simulink model "coherent_demodulation"  (R2018b)
settings: Solver=VariableStepAuto  StartTime=0.0  StopTime=1  RelTol=1e-3
libraries: dsparch4 x2, commchan3 x1
settings Model: Creator=sangh  LastModifiedBy=sangh

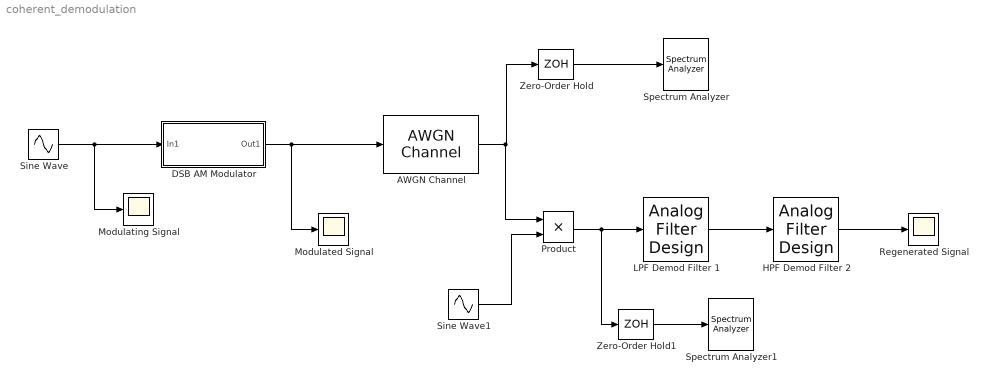
== system coherent_demodulation ==
  AWGN Channel : commchan3/AWGN Channel  InputProcessing=Columns as channels (frame based)  seed=randseed  noiseMode=Variance from mask  EbNodB=10  EsNodB=10  SNRdB=10  bitsPerSym=1  Ps=1  Tsym=1  variance=0
  DSB AM Modulator : Subsystem
  HPF Demod Filter 2 : dsparch4/Analog Filter Design  method=Butterworth  filttype=Highpass  N=8  Wlo=200*pi  Whi=80  Rp=2  Rs=40
  LPF Demod Filter 1 : dsparch4/Analog Filter Design  method=Butterworth  filttype=Lowpass  N=8  Wlo=1500*pi  Whi=80  Rp=2  Rs=40
  Modulated Signal : Scope
  Modulating Signal : Scope
  Product : Product
  Regenerated Signal : Scope
  Sine Wave : Sin  Frequency=2*pi*500  SampleTime=0.25e-6
  Sine Wave1 : Sin  Frequency=2*pi*20e3  SampleTime=0.25e-6
  Spectrum Analyzer : SpectrumAnalyzer
  Spectrum Analyzer1 : SpectrumAnalyzer
  Zero-Order Hold : ZeroOrderHold  SampleTime=-1
  Zero-Order Hold1 : ZeroOrderHold  SampleTime=-1
  wires:
  AWGN Channel/1 -> Product/1, Zero-Order Hold/1
  Sine Wave/1 -> Modulating Signal/1, DSB AM Modulator/1(In1)
  DSB AM Modulator/1(Out1) -> AWGN Channel/1, Modulated Signal/1
  Zero-Order Hold/1 -> Spectrum Analyzer/1
  Sine Wave1/1 -> Product/2
  Product/1 -> Zero-Order Hold1/1, LPF Demod Filter 1/1
  LPF Demod Filter 1/1 -> HPF Demod Filter 2/1
  Zero-Order Hold1/1 -> Spectrum Analyzer1/1
  HPF Demod Filter 2/1 -> Regenerated Signal/1

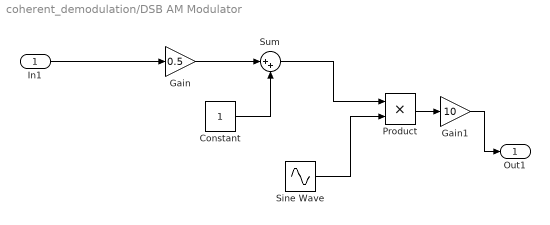
== system coherent_demodulation/DSB AM Modulator ==
  In1 : Inport
  Constant : Constant
  Gain : Gain  Gain=0.5
  Gain1 : Gain  Gain=10
  Product : Product
  Sine Wave : Sin  Frequency=2*pi*20e3  SampleTime=0.25e-6
  Sum : Sum  Inputs=|++
  Out1 : Outport
  wires:
  In1/1 -> Gain/1
  Gain/1 -> Sum/1
  Constant/1 -> Sum/2
  Sine Wave/1 -> Product/2
  Sum/1 -> Product/1
  Product/1 -> Gain1/1
  Gain1/1 -> Out1/1
